simulink model "RefModel_compass_out"  (R2019b)
settings: Solver=FixedStepDiscrete  StartTime=0.0  StopTime=120  FixedStep=0.004  RelTol=1e-3
values from neighbouring files (symbols this model uses):
  ax = double(typecast(uint8(temp),'single')')/1*1.0000000000    [V1000_decode_auto.m]
  ay = double(typecast(uint8(temp),'single')')/1*1.0000000000    [V1000_decode_auto.m]
  az = double(typecast(uint8(temp),'single')')/1*1.0000000000    [V1000_decode_auto.m]
  gx = double(typecast(uint8(temp),'single')')/1*1.0000000000    [V1000_decode_auto.m]
  gy = double(typecast(uint8(temp),'single')')/1*1.0000000000    [V1000_decode_auto.m]
  gz = double(typecast(uint8(temp),'single')')/1*1.0000000000    [V1000_decode_auto.m]
undefined symbols (not defined in the file or in its folder): ax_f, ay_f, az_f, mag2_xx, mag2_yx, mag2_zx, rtU_MagYaw_acc_0, rtU_MagYaw_acc_1, rtU_MagYaw_acc_2, rtU_MagYaw_out, time_algo, time_imu, time_mag, time_mag_yaw, time_ublox, ublox_lat, ublox_lon
libraries: simulink x1, aerolibgravity2 x1
settings Model: PauseTimes=30  Creator=sl  LastModifiedBy=a4327
settings OptimizationCC: DefaultParameterBehavior=Inlined  UseDivisionForNetSlopeComputation=on  GainParamInheritBuiltInType=on  UseFloatMulNetSlope=on  InlineInvariantSignals=on  PassReuseOutputArgsAs=Individual arguments  ZeroExternalMemoryAtStartup=off  ZeroInternalMemoryAtStartup=off  NoFixptDivByZeroProtection=on  EfficientFloat2IntCast=on  LifeSpan=1  OptimizeBlockOrder=speed  DifferentSizesBufferReuse=on  EfficientTunableParamExpr=on
settings DebuggingCC: ParameterTunabilityLossMsg=error  ArithmeticOperatorsInVariantConditions=warning
settings HardwareCC: ProdBitPerPointer=32  ProdBitPerSizeT=32  ProdBitPerPtrDiffT=32  ProdLargestAtomicFloat=None  ProdWordSize=32  ProdLongLongMode=on  ProdHWDeviceType=Custom Processor->Custom Processor
settings SFSimCC: MATLABDynamicMemAlloc=off  CustomCodeUndefinedFunction=UseInterfaceOnly
settings RTWCC: SystemTargetFile=ert.tlc  TemplateMakefile=ert_default_tmf  GenerateReport=on  IncludeHyperlinkInReport=on  LaunchReport=on  GenerateTraceInfo=on  GenerateTraceReport=on  GenerateTraceReportSl=on  GenerateTraceReportSf=on  GenerateTraceReportEml=on  GenerateCodeMetricsReport=on
settings CodeAppCC: ForceParamTrailComments=on  IgnoreCustomStorageClasses=off  OperatorAnnotations=on  SimulinkDataObjDesc=on  SFDataObjDesc=on  CustomSymbolStrGlobalVar=rt$N$M  CustomSymbolStrType=$N$M  CustomSymbolStrFcn=$N$M$F  CustomSymbolStrMacro=$N$M  InsertBlockDesc=on
settings ERTTargetCC: TargetLangStandard=C99 (ISO)  GenerateSampleERTMain=on  IncludeMdlTerminateFcn=off  CombineSignalStateStructs=on  SupportComplex=off  SupportContinuousTime=on  SupportNonInlinedSFcns=on  InlinedParameterPlacement=NonHierarchical  ERTCustomFileTemplate=example_file_process.tlc  ERTFilePackagingFormat=CompactWithDataFile

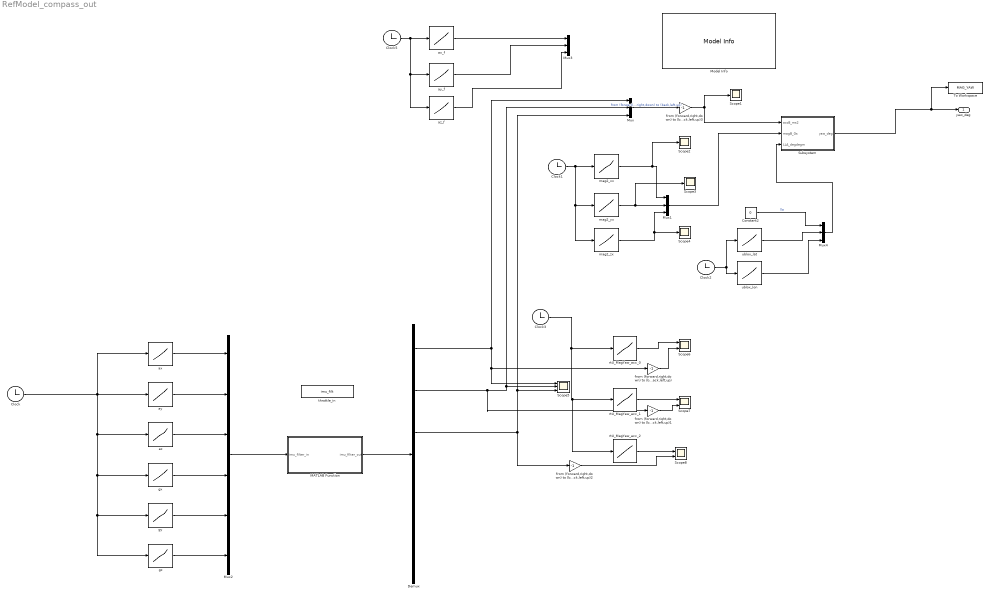
== system RefModel_compass_out ==
  Clock{,1..3,5} (5 alike) : Clock
  Constant2 : Constant  Value=0
  Demux : Demux  Outputs=6
  MATLAB Function : MATLAB Function  TreatAsAtomicUnit=on
  Model Info : simulink/Model-Wide Utilities/Model Info  Frame=on  DisplayStringWithTags=|  HorizontalTextAlignment=Left  LeftAlignmentValue=0.02
      | %<ModelVersion>
      | %<LastModificationDate>
      | 
      | Body Coordinate: forward - right - down
      | Navigation Coordinate: NED
      | 
      | input:
      | 	accB_ms2:  1x3  m/s^2
      | 	magB_Gs:   1x3  Gs
      | 	LLA_degdegm(lat,lon,height): 1x3 deg,deg,m  
      | output:
      | 	yaw_deg: 1x1 deg
  Mux{,1,3..4} (4 alike) : Mux  Inputs=3
  Mux2 : Mux  Inputs=6
  Scope{1..4} (4 alike) : Scope
  Scope5 : Scope  NumInputPorts=3
  Scope6 : Scope  NumInputPorts=2
  Scope7 : Scope  NumInputPorts=2
  Scope8 : Scope  NumInputPorts=2
  Subsystem : Subsystem
  To Workspace : ToWorkspace  VariableName=MAG_YAW  SampleTime=-1
  ax : Lookup_n-D  NumberOfTableDimensions=1  BreakpointsForDimension1=time_imu  Table=ax  InternalRulePriority=Speed  RndMeth=Simplest  InputSameDT=on
  ax_f : Lookup_n-D  NumberOfTableDimensions=1  BreakpointsForDimension1=time_algo  Table=ax_f  InternalRulePriority=Speed  RndMeth=Simplest  InputSameDT=on
  ay : Lookup_n-D  NumberOfTableDimensions=1  BreakpointsForDimension1=time_imu  Table=ay  InternalRulePriority=Speed  RndMeth=Simplest  InputSameDT=on
  ay_f : Lookup_n-D  NumberOfTableDimensions=1  BreakpointsForDimension1=time_algo  Table=ay_f  InternalRulePriority=Speed  RndMeth=Simplest  InputSameDT=on
  az : Lookup_n-D  NumberOfTableDimensions=1  BreakpointsForDimension1=time_imu  Table=az  InternalRulePriority=Speed  RndMeth=Simplest  InputSameDT=on
  az_f : Lookup_n-D  NumberOfTableDimensions=1  BreakpointsForDimension1=time_algo  Table=az_f  InternalRulePriority=Speed  RndMeth=Simplest  InputSameDT=on
  from (forward,right,down) to (back,left,up){,1..3} (4 alike) : Gain  Gain=-1
  gx : Lookup_n-D  NumberOfTableDimensions=1  BreakpointsForDimension1=time_imu  Table=gx  InternalRulePriority=Speed  RndMeth=Simplest  InputSameDT=on
  gy : Lookup_n-D  NumberOfTableDimensions=1  BreakpointsForDimension1=time_imu  Table=gy  InternalRulePriority=Speed  RndMeth=Simplest  InputSameDT=on
  gz : Lookup_n-D  NumberOfTableDimensions=1  BreakpointsForDimension1=time_imu  Table=gz  InternalRulePriority=Speed  RndMeth=Simplest  InputSameDT=on
  mag2_xx : Lookup_n-D  NumberOfTableDimensions=1  BreakpointsForDimension1=time_mag  Table=mag2_xx  InternalRulePriority=Speed  RndMeth=Simplest  InputSameDT=on
  mag2_yx : Lookup_n-D  NumberOfTableDimensions=1  BreakpointsForDimension1=time_mag  Table=mag2_yx  InternalRulePriority=Speed  RndMeth=Simplest  InputSameDT=on
  mag2_zx : Lookup_n-D  NumberOfTableDimensions=1  BreakpointsForDimension1=time_mag  Table=mag2_zx  InternalRulePriority=Speed  RndMeth=Simplest  InputSameDT=on
  rtU_MagYaw_acc_0 : Lookup_n-D  NumberOfTableDimensions=1  BreakpointsForDimension1=time_mag_yaw  Table=rtU_MagYaw_acc_0  InternalRulePriority=Speed  RndMeth=Simplest  InputSameDT=on
  rtU_MagYaw_acc_1 : Lookup_n-D  NumberOfTableDimensions=1  BreakpointsForDimension1=time_mag_yaw  Table=rtU_MagYaw_acc_1  InternalRulePriority=Speed  RndMeth=Simplest  InputSameDT=on
  rtU_MagYaw_acc_2 : Lookup_n-D  NumberOfTableDimensions=1  BreakpointsForDimension1=time_mag_yaw  Table=rtU_MagYaw_acc_2  InternalRulePriority=Speed  RndMeth=Simplest  InputSameDT=on
  throttle_in : DataStoreMemory  DataStoreName=imu_filt  ReadBeforeWriteMsg=warning  WriteAfterWriteMsg=warning  WriteAfterReadMsg=warning  InitialValue=imu_filt  VectorParams1D=off  ShowAdditionalParam=off  OutDataTypeStr=double
  ublox_lat : Lookup_n-D  NumberOfTableDimensions=1  BreakpointsForDimension1=time_ublox  Table=ublox_lat  InternalRulePriority=Speed  RndMeth=Simplest  InputSameDT=on
  ublox_lon : Lookup_n-D  NumberOfTableDimensions=1  BreakpointsForDimension1=time_ublox  Table=ublox_lon  InternalRulePriority=Speed  RndMeth=Simplest  InputSameDT=on
  yaw_deg : Outport
  wires:
  Mux/1 -> from (forward,right,down) to (back,left,up)3/1  "from (forward,right,down) to (back,left,up)"
  Subsystem/1(yaw_deg) -> To Workspace/1, yaw_deg/1
  Clock5/1 -> ax_f/1, ay_f/1, az_f/1
  Clock1/1 -> mag2_zx/1, mag2_yx/1, mag2_xx/1
  gy/1 -> Mux2/5
  gz/1 -> Mux2/6
  ay/1 -> Mux2/2
  Mux2/1 -> MATLAB Function/1(imu_filter_in)
  ax/1 -> Mux2/1
  az/1 -> Mux2/3
  Clock/1 -> gz/1, gy/1, gx/1, az/1, ax/1, ay/1
  gx/1 -> Mux2/4
  MATLAB Function/1(imu_filter_out) -> Demux/1
  mag2_yx/1 -> Scope3/1, Mux1/2
  mag2_xx/1 -> Scope2/1, Mux1/1
  mag2_zx/1 -> Scope4/1, Mux1/3
  Demux/1 -> from (forward,right,down) to (back,left,up)/1, Scope5/1, Mux/1
  Demux/2 -> from (forward,right,down) to (back,left,up)1/1, Scope5/2, Mux/2
  Demux/3 -> from (forward,right,down) to (back,left,up)2/1, Scope5/3, Mux/3
  Mux1/1 -> Subsystem/2(magB_Gs)
  ax_f/1 -> Mux3/1
  ay_f/1 -> Mux3/2
  az_f/1 -> Mux3/3
  Constant2/1 -> Mux4/1  "lla"
  Clock2/1 -> ublox_lon/1, ublox_lat/1
  Mux4/1 -> Subsystem/3(LLA_degdegm)
  ublox_lat/1 -> Mux4/2
  ublox_lon/1 -> Mux4/3
  Clock3/1 -> rtU_MagYaw_acc_2/1, rtU_MagYaw_acc_1/1, rtU_MagYaw_acc_0/1
  rtU_MagYaw_acc_0/1 -> Scope6/1
  rtU_MagYaw_acc_1/1 -> Scope7/1
  rtU_MagYaw_acc_2/1 -> Scope8/1
  from (forward,right,down) to (back,left,up)/1 -> Scope6/2
  from (forward,right,down) to (back,left,up)1/1 -> Scope7/2
  from (forward,right,down) to (back,left,up)2/1 -> Scope8/2
  from (forward,right,down) to (back,left,up)3/1 -> Scope1/1, Subsystem/1(accB_ms2)

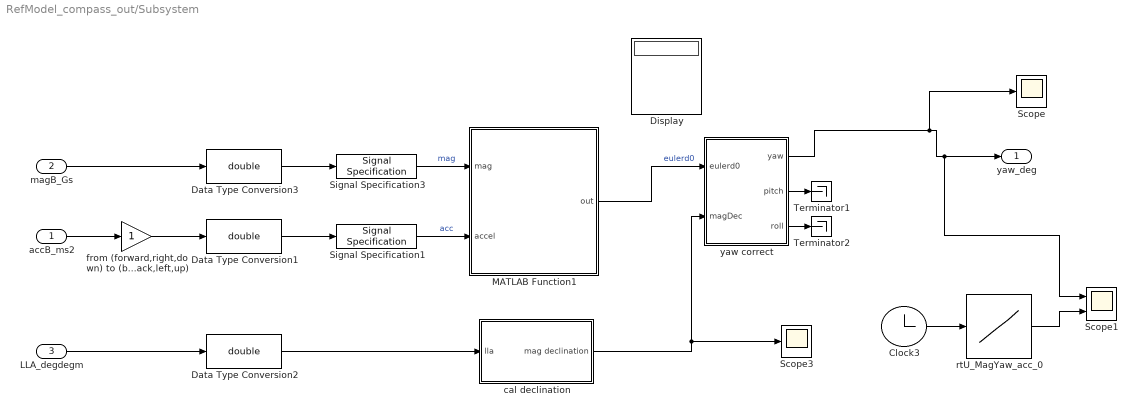
== system RefModel_compass_out/Subsystem ==
  accB_ms2 : Inport  PortDimensions=[1,3]
  magB_Gs : Inport  Port=2  PortDimensions=[1,3]
  LLA_degdegm : Inport  Port=3  PortDimensions=[1,3]
  Clock3 : Clock
  Data Type Conversion1 : DataTypeConversion  OutDataTypeStr=double
  Data Type Conversion2 : DataTypeConversion  OutDataTypeStr=double
  Data Type Conversion3 : DataTypeConversion  OutDataTypeStr=double
  Display : Display
  MATLAB Function1 : MATLAB Function  TreatAsAtomicUnit=on
  Scope : Scope
  Scope1 : Scope  NumInputPorts=2
  Scope3 : Scope
  Signal Specification1 : SignalSpecification  Dimensions=[1,3]
  Signal Specification3 : SignalSpecification  Dimensions=[1,3]
  Terminator1 : Terminator
  Terminator2 : Terminator
  cal declination : Subsystem
  from (forward,right,down) to (back,left,up) : Gain
  rtU_MagYaw_acc_0 : Lookup_n-D  NumberOfTableDimensions=1  BreakpointsForDimension1=time_mag_yaw  Table=rtU_MagYaw_out  InternalRulePriority=Speed  RndMeth=Simplest  InputSameDT=on
  yaw correct : Subsystem
  yaw_deg : Outport
  wires:
  from (forward,right,down) to (back,left,up)/1 -> Data Type Conversion1/1
  Signal Specification3/1 -> MATLAB Function1/1(mag)  "mag"
  yaw correct/2(pitch) -> Terminator1/1
  Data Type Conversion1/1 -> Signal Specification1/1
  Data Type Conversion3/1 -> Signal Specification3/1
  magB_Gs/1 -> Data Type Conversion3/1
  accB_ms2/1 -> from (forward,right,down) to (back,left,up)/1
  yaw correct/3(roll) -> Terminator2/1
  Signal Specification1/1 -> MATLAB Function1/2(accel)  "acc"
  cal declination/1(mag declination) -> yaw correct/2(magDec), Scope3/1
  Data Type Conversion2/1 -> cal declination/1(lla)
  LLA_degdegm/1 -> Data Type Conversion2/1
  MATLAB Function1/1(out) -> yaw correct/1(eulerd0)  "eulerd0"
  yaw correct/1(yaw) -> Scope/1, Scope1/1, yaw_deg/1
  Clock3/1 -> rtU_MagYaw_acc_0/1
  rtU_MagYaw_acc_0/1 -> Scope1/2

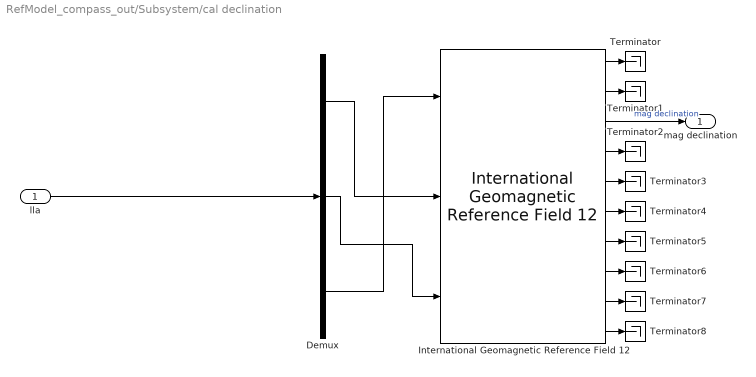
== system RefModel_compass_out/Subsystem/cal declination ==
  lla : Inport
  Demux : Demux  Outputs=3
  International Geomagnetic Reference Field 12 : aerolibgravity2/International Geomagnetic Reference Field 12  units=Metric (MKS)  time_in=off  month=December  day=20  year=2019  action=None  sv_out=on
      settings: SourceProductName=Aerospace Blockset  SourceProductBaseCode=AE
  Terminator{,1..8} (9 alike) : Terminator
  mag declination : Outport
  wires:
  Demux/3 -> International Geomagnetic Reference Field 12/1
  Demux/1 -> International Geomagnetic Reference Field 12/2
  International Geomagnetic Reference Field 12/9 -> Terminator7/1
  International Geomagnetic Reference Field 12/10 -> Terminator8/1
  International Geomagnetic Reference Field 12/4 -> Terminator2/1
  International Geomagnetic Reference Field 12/1 -> Terminator/1
  Demux/2 -> International Geomagnetic Reference Field 12/3
  International Geomagnetic Reference Field 12/2 -> Terminator1/1
  International Geomagnetic Reference Field 12/3 -> mag declination/1  "mag declination"
  International Geomagnetic Reference Field 12/5 -> Terminator3/1
  International Geomagnetic Reference Field 12/6 -> Terminator4/1
  International Geomagnetic Reference Field 12/8 -> Terminator6/1
  International Geomagnetic Reference Field 12/7 -> Terminator5/1
  lla/1 -> Demux/1

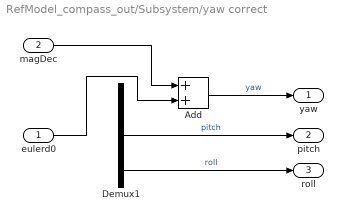
== system RefModel_compass_out/Subsystem/yaw correct ==
  eulerd0 : Inport
  magDec : Inport  Port=2
  Add : Sum
  Demux1 : Demux  Outputs=3
  yaw : Outport
  pitch : Outport  Port=2
  roll : Outport  Port=3
  wires:
  magDec/1 -> Add/1
  Demux1/2 -> pitch/1  "pitch"
  Demux1/3 -> roll/1  "roll"
  eulerd0/1 -> Add/2
  Add/1 -> yaw/1  "yaw"

== matlab function RefModel_compass_out/MATLAB Function ==
  data: imu_filter_in input; imu_filter_out output; imu_filt data_store_memory
function imu_filter_out = imu_filter(imu_filter_in)
% ftz.num{1:end}
% ftz.den{1:end}
% persistent
persistent imu_filter_temp
persistent dt
global imu_filt
    if isempty(imu_filter_temp)
        imu_filter_temp = zeros(6,1);
    end
    
   if isempty(dt)
        dt = 0.004;
    end

  rc=1/(2*pi*imu_filt);
  alpha=dt/(dt+rc);
  imu_filter_temp=imu_filter_temp+(imu_filter_in-imu_filter_temp)*alpha;
  imu_filter_out=imu_filter_temp;  
    
%     
% 
% imu_filter_in_buff(1,:)=imu_filter_in_buff(2,:);
% imu_filter_in_buff(2,:)=imu_filter_in_buff(3,:);
% imu_filter_in_buff(3,:)=imu_filter_in;
% imu_filter_out_buff(1,:)=imu_filter_out_buff(2,:);
% imu_filter_out_buff(2,:)=imu_filter_out_buff(3,:);
% % imu_filter_out=imu_filter_in_buff(3,:)*0.1287+imu_filter_in_buff(2,:)*0.2574+imu_filter_in_buff(1,:)*0.1287-imu_filter_out_buff(2,:)*- 0.7613-imu_filter_out_buff(1,:)*0.276;
% imu_filter_out=imu_filter_in_buff(3,:)*0.008771+imu_filter_in_buff(2,:)*0.01754+imu_filter_in_buff(1,:)*0.008771-imu_filter_out_buff(2,:)*- 1.718-imu_filter_out_buff(1,:)*0.7533;
% % imu_filter_out=imu_filter_in_buff(3,:)*0.003613+imu_filter_in_buff(2,:)*0.007225+imu_filter_in_buff(1,:)*0.003613-imu_filter_out_buff(2,:)*- 1.823-imu_filter_out_buff(1,:)*0.8374;
% 
% imu_filter_out_buff(3,:)=imu_filter_out;

== matlab function RefModel_compass_out/Subsystem/MATLAB Function1 ==
  data: mag input; accel input; out output
function out  = compass(mag,accel)
    quat0 = zeros(1,4);
    eulerd0 = zeros(1,3);
    temp=ecompass(accel,mag);
    quat0 = compact(temp);
%      eulerd0 = eulerd(quat0);
     eulerd0 = to_euler(quat0);
    out=eulerd0(3);
    
    
%     out=atan2(mag(2),mag(1));
%     if out<-0
%     out=out+2*pi;
%     end
    out=out*180/pi;
end


function eout = eulerd(quat)
% rotate 'ZYX'
qa = quat(1);
qb = quat(2);
qc = quat(3);
qd = quat(4);
the1 = 1;
the2 = 2;

tmp = qb.*qd.*the2 - qa.*qc.*the2;
if tmp > the1
    tmp = the1;
elseif tmp < -the1
    tmp = -the1;
end
% tmp(tmp > the1) = the1;
% tmp(tmp < -the1) = -the1;
b = -asin(tmp);
a = atan2((qa.*qd.*the2 + qb.*qc.*the2),(qa.^2.*the2 - the1 + qb.^2.*the2));
c = atan2((qa.*qb.*the2 + qc.*qd.*the2),(qa.^2.*the2 - the1 + qd.^2.*the2));
eout = [a b c];
end
% 
% function [eulerd0,quat0] = compass(i,accel,mag,imuUpdateFs,magUpdateFs)
%     fs = imuUpdateFs;
%     quat0 = zeros(1,4);
%     eulerd0 = zeros(1,3);
%     if rem(i,fs/magUpdateFs) == 0 && i ~= 1
%         quat0 = compact(ecompass(accel,mag));
%         eulerd0 = eulerd(quat0);
%     end
% end
